simulink model "simulink_problem17"  (R2019b)
settings: Solver=VariableStepAuto  StartTime=0.0  StopTime=8  RelTol=1e-3
values from neighbouring files (symbols this model uses):
  A1 = KT    (= 0.17)    [problem15.m]    (also in problem16.m; problem17.m; problem18.m; problem4.m = Q1/T)
  A2 = KT    (= 0.17)    [problem15.m]    (also in problem16.m; problem17.m; problem18.m; problem4.m = Q2/T)
  A3 = KT    (= 0.17)    [problem15.m]    (also in problem16.m; problem17.m; problem18.m; problem4.m = Q3/T)
  A4 = KT    (= 0.17)    [problem15.m]    (also in problem16.m; problem17.m; problem18.m; problem4.m = Q4/T)
  a4 = 0.98    [problem17.m]    (also in problem18.m; problem20.m; problem21.m; problem7.m)
  C1 = n^2 * den1    [problem15.m]    (also in problem16.m = n^2 * d1; problem17.m; problem18.m)
  C2 = n^2 * den2    [problem15.m]    (also in problem16.m = n^2 * d2; problem17.m; problem18.m)
  C3 = n^2 * den3    [problem15.m]    (also in problem16.m = n^2 * d3; problem17.m; problem18.m)
  C4 = n^2 * den4    [problem15.m]    (also in problem16.m = n^2 * d4; problem17.m; problem18.m)
  d1 = [JM (f_eff + KT * KD1) (KT * KP1)]    [problem12.m]    (also in problem16.m = [J_eff(1)  (f_eff + KT*KD1)  KT*KP1  KT*KI]; problem17.m = 1.5; problem18.m = 1.5; problem20.m = 1.5)
  den1 = [J_eff(1)  (f_eff + KT*KD1)  KT*KP1  KT*KI]    [problem15.m]    (also in problem17.m = [J_eff(1)  (f_eff + k_T*KD1)  k_T*KP1  k_T*KI]; problem18.m = [J_eff(1)  (f_eff + k_T*KD1)  k_T*KP1  k_T*KI])
  den2 = [J_eff(2)  (f_eff + KT*KD2)  KT*KP2  KT*KI]    [problem15.m]    (also in problem17.m = [J_eff(2)  (f_eff + k_T*KD2)  k_T*KP2  k_T*KI]; problem18.m = [J_eff(2)  (f_eff + k_T*KD2)  k_T*KP2  k_T*KI])
  den3 = [J_eff(3)  (f_eff + KT*KD3)  KT*KP3  KT*KI]    [problem15.m]    (also in problem17.m = [J_eff(3)  (f_eff + k_T*KD3)  k_T*KP3  k_T*KI]; problem18.m = [J_eff(3)  (f_eff + k_T*KD3)  k_T*KP3  k_T*KI])
  den4 = [J_eff(4)  (f_eff + KT*KD4)  KT*KP4  KT*KI]    [problem15.m]    (also in problem17.m = [J_eff(4)  (f_eff + k_T*KD4)  k_T*KP4  k_T*KI]; problem18.m = [J_eff(4)  (f_eff + k_T*KD4)  k_T*KP4  k_T*KI])
  num1 = KT * [KD1  KP1  KI]    [problem15.m]    (also in problem17.m = k_T * [KD1  KP1  KI]; problem18.m = k_T * [KD1  KP1  KI])
  num2 = KT * [KD2  KP2  KI]    [problem15.m]    (also in problem17.m = k_T * [KD2  KP2  KI]; problem18.m = k_T * [KD2  KP2  KI])
  num3 = KT * [KD3  KP3  KI]    [problem15.m]    (also in problem17.m = k_T * [KD3  KP3  KI]; problem18.m = k_T * [KD3  KP3  KI])
  num4 = KT * [KD4  KP4  KI]    [problem15.m]    (also in problem17.m = k_T * [KD4  KP4  KI]; problem18.m = k_T * [KD4  KP4  KI])
settings Model: Creator=ben  LastModifiedBy=ben

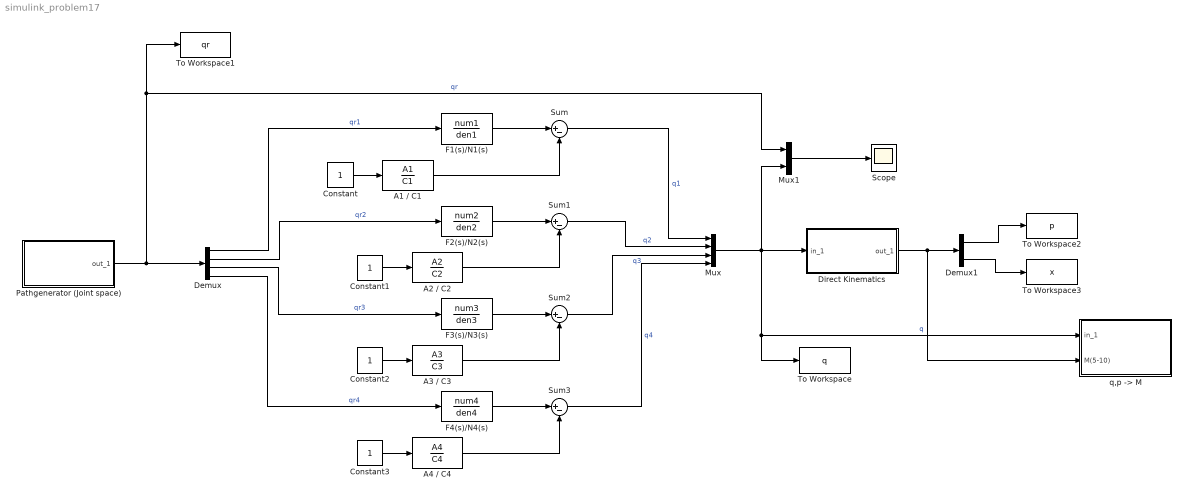
== system simulink_problem17 ==
  A1 / C1 : TransferFcn  Numerator=A1  Denominator=C1
  "A2 / C2 " : TransferFcn  Numerator=A2  Denominator=C2
  "A3 / C3 " : TransferFcn  Numerator=A3  Denominator=C3
  A4 / C4 : TransferFcn  Numerator=A4  Denominator=C4
  Constant{,1..3} (4 alike) : Constant
  Demux : Demux
  Demux1 : Demux  Outputs=2
  Direct Kinematics : Subsystem
      mask Display: disp('Alto-Robot')
  F1(s)/N1(s) : TransferFcn  Numerator=num1  Denominator=den1
  F2(s)/N2(s) : TransferFcn  Numerator=num2  Denominator=den2
  F3(s)/N3(s) : TransferFcn  Numerator=num3  Denominator=den3
  F4(s)/N4(s) : TransferFcn  Numerator=num4  Denominator=den4
  Mux : Mux
  Mux1 : Mux  Inputs=2
  Pathgenerator (Joint space) : Subsystem
      mask Display: disp('Alto-Robot\n path -> q')
  Scope : Scope
  Sum{,1..3} (4 alike) : Sum  Inputs=|+-
  To Workspace : ToWorkspace  VariableName=q  SaveFormat=Timeseries  SampleTime=-1
  To Workspace1 : ToWorkspace  VariableName=qr  SaveFormat=Timeseries  SampleTime=-1
  To Workspace2 : ToWorkspace  VariableName=p  SaveFormat=Timeseries  SampleTime=-1
  To Workspace3 : ToWorkspace  VariableName=x  SaveFormat=Timeseries  SampleTime=-1
  "q,p -> M" : Subsystem
      mask Display: disp('Save to vis4link')
  wires:
  F1(s)/N1(s)/1 -> Sum/1
  Sum/1 -> Mux/1  "q1"
  Sum1/1 -> Mux/2  "q2"
  F2(s)/N2(s)/1 -> Sum1/1
  Sum2/1 -> Mux/3  "q3"
  F3(s)/N3(s)/1 -> Sum2/1
  Sum3/1 -> Mux/4  "q4"
  F4(s)/N4(s)/1 -> Sum3/1
  Demux/1 -> F1(s)/N1(s)/1  "qr1"
  Demux/2 -> F2(s)/N2(s)/1  "qr2"
  Demux/3 -> F3(s)/N3(s)/1  "qr3"
  Demux/4 -> F4(s)/N4(s)/1  "qr4"
  Constant/1 -> A1 / C1/1
  A1 / C1/1 -> Sum/2
  Constant1/1 -> "A2 / C2 "/1
  "A2 / C2 "/1 -> Sum1/2
  Constant2/1 -> "A3 / C3 "/1
  "A3 / C3 "/1 -> Sum2/2
  Constant3/1 -> A4 / C4/1
  A4 / C4/1 -> Sum3/2
  Pathgenerator (Joint space)/1(out_1) -> To Workspace1/1, Mux1/1, Demux/1  "qr"
  Mux/1 -> "q,p -> M"/1(in_1), To Workspace/1, Mux1/2, Direct Kinematics/1(in_1)  "q"
  Mux1/1 -> Scope/1
  Direct Kinematics/1(out_1) -> "q,p -> M"/2(M(5-10)), Demux1/1
  Demux1/1 -> To Workspace2/1
  Demux1/2 -> To Workspace3/1

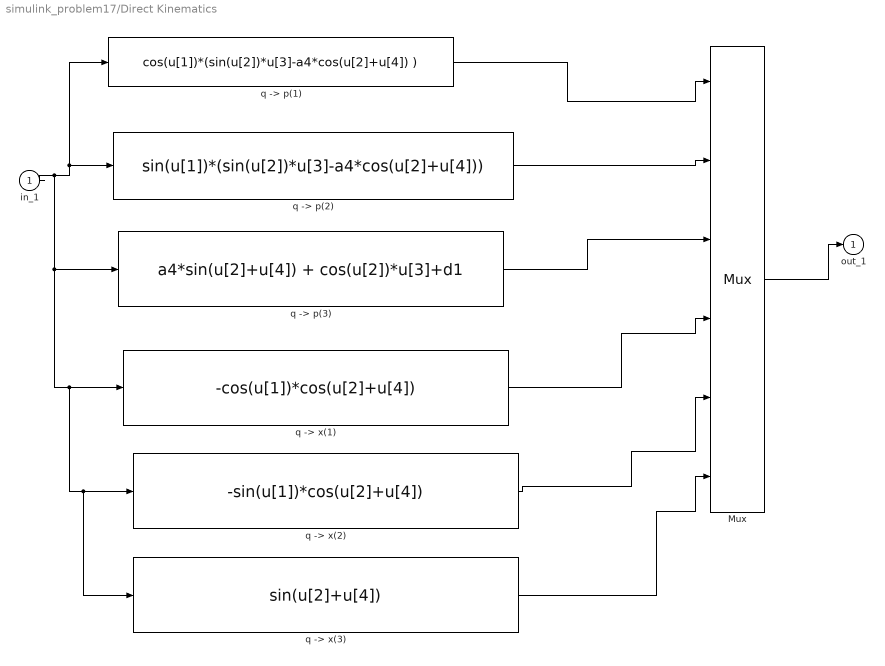
== system simulink_problem17/Direct Kinematics ==
  in_1 : Inport
  Mux : Mux  Inputs=6
  "q -> p(1)" : Fcn  Expr=cos(u[1])*(sin(u[2])*u[3]-a4*cos(u[2]+u[4]) )
  "q -> p(2)" : Fcn  Expr=sin(u[1])*(sin(u[2])*u[3]-a4*cos(u[2]+u[4]))
  "q -> p(3)" : Fcn  Expr=a4*sin(u[2]+u[4]) + cos(u[2])*u[3]+d1
  "q -> x(1)" : Fcn  Expr=-cos(u[1])*cos(u[2]+u[4])
  "q -> x(2)" : Fcn  Expr=-sin(u[1])*cos(u[2]+u[4])
  "q -> x(3)" : Fcn  Expr=sin(u[2]+u[4])
  out_1 : Outport  InitialOutput=0  VectorParamsAs1DForOutWhenUnconnected=off
  wires:
  Mux/1 -> out_1/1
  in_1/1 -> "q -> x(3)"/1, "q -> x(2)"/1, "q -> x(1)"/1, "q -> p(3)"/1, "q -> p(2)"/1, "q -> p(1)"/1
  "q -> x(3)"/1 -> Mux/6
  "q -> x(2)"/1 -> Mux/5
  "q -> x(1)"/1 -> Mux/4
  "q -> p(1)"/1 -> Mux/1
  "q -> p(2)"/1 -> Mux/2
  "q -> p(3)"/1 -> Mux/3

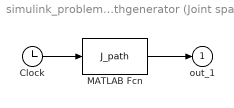
== system simulink_problem17/Pathgenerator (Joint space) ==
  Clock : Clock
  MATLAB Fcn : MATLABFcn  MATLABFcn=J_path  OutputDimensions=4
  out_1 : Outport  VectorParamsAs1DForOutWhenUnconnected=off
  wires:
  MATLAB Fcn/1 -> out_1/1
  Clock/1 -> MATLAB Fcn/1

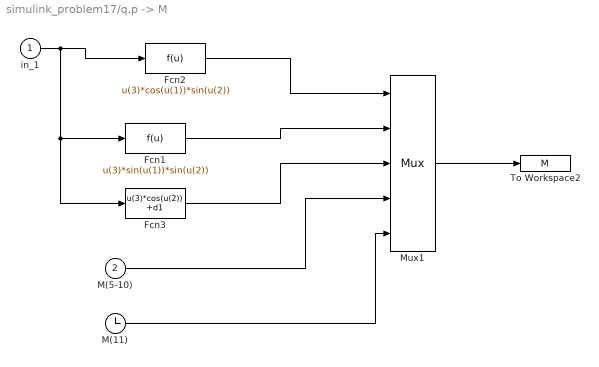
== system simulink_problem17/q,p -> M ==
  in_1 : Inport
  M(5-10) : Inport  Port=2
  Fcn1 : Fcn  Expr=u(3)*sin(u(1))*sin(u(2))
  Fcn2 : Fcn  Expr=u(3)*cos(u(1))*sin(u(2))
  Fcn3 : Fcn  Expr=u(3)*cos(u(2)) +d1
  M(11) : Clock
  Mux1 : Mux  Inputs=[1 1 1 6 1]
  To Workspace2 : ToWorkspace  VariableName=M
      settings: MaxDataPoints=100000
  wires:
  M(11)/1 -> Mux1/5
  M(5-10)/1 -> Mux1/4
  Fcn3/1 -> Mux1/3
  Fcn1/1 -> Mux1/2
  Fcn2/1 -> Mux1/1
  in_1/1 -> Fcn3/1, Fcn1/1, Fcn2/1
  Mux1/1 -> To Workspace2/1
